simulink model "LineFollowing"  (R2013a)
settings: Solver=ode4  SolverMode=SingleTasking  StartTime=0.0  StopTime=pi  RelTol=1e-3
model workspace (MAT data in the model file):
  axleLength = Simulink.Parameter
  axleLength.Value = 9.8
  axleLength.Description = 'Distance between tire contact points
    | of the two wheels/treads
    | in units of centimeters.'
  axleLength.DataType = 'auto'
  commandPercmPerSecond = Simulink.Parameter
  commandPercmPerSecond.Value = 3.9547
  commandPercmPerSecond.Description = 'Convert units of ''command'' 
    | to units of ''cm/s''.
    | 
    | ''command'' is a value in the range [-256, 255].'
  commandPercmPerSecond.DataType = 'auto'
  symmetrizeMotors = Simulink.Parameter
  symmetrizeMotors.Value = 1
  symmetrizeMotors.Description = 'Scale one of the motor commands down 
    | (not up) to balance the motors. 
    | Once balanced, a value of x sent to either
    | motor will produce the same rate of rotation
    | in both motors.'
  symmetrizeMotors.DataType = 'auto'
  sampleTime = Simulink.Parameter
  sampleTime.Value = 0.01
  sampleTime.Description = 'Sample time (in seconds) of the trajectory simulator.'
  sampleTime.DataType = 'auto'
  commandThreshold = Simulink.Parameter
  commandThreshold.Value = 31.875
  commandThreshold.DataType = 'auto'
  plotRange = Simulink.Parameter
  plotRange.Value = 50
  plotRange.Description = 'Range of trajectory plot in units
    | of centimeters.'
  plotRange.DataType = 'auto'
libraries: ZumoBotLib x2, simulink x1
settings Model: ExtModeTrigDuration=2  Creator=pkasseba  LastModifiedBy=adesai
settings DataIOCC: SignalLoggingSaveFormat=ModelDataLogs
settings OptimizationCC: OptimizeModelRefInitCode=on  LifeSpan=1
settings DebuggingCC: SolverPrmCheckMsg=none  MultiTaskDSMMsg=warning  MultiTaskCondExecSysMsg=none  StateNameClashWarn=none  StrictBusMsg=None
settings HardwareCC: ProdBitPerInt=16  ProdBitPerPointer=8  ProdIntDivRoundTo=Zero  ProdEndianess=LittleEndian  ProdWordSize=8  ProdHWDeviceType=Atmel->AVR
settings RTWCC: SystemTargetFile=realtime.tlc  GenerateMakefile=off  TemplateMakefile=realtime.tmf  Description=Run on Target Hardware  RTWVerbose=off  ProcessScript=realtime_make_rtw_hook  IncludeERTFirstTime=on
settings STFCustomTargetCC: TargetLibSuffix=.a  GenerateSampleERTMain=on  ERTCustomFileBanners=on  SupportNonInlinedSFcns=off  SupportVariableSizeSignals=on  MATLABClassNameForMDSCustomization=Simulink.SoftwareTarget.ERTCustomization  SystemTargetFile=realtime.tlc
settings ERTTargetCC: ParMdlRefBuildCompliant=off  CompOptLevelCompliant=off  ConcurrentExecutionCompliant=off  CombineOutputUpdateFcns=off  ERTFirstTimeCompliant=off  SupportContinuousTime=on  SupportVariableSizeSignals=on  ModelStepFunctionPrototypeControlCompliant=off  CPPClassGenCompliant=off  ExtModeTransport=3  ExtModeMexFile=ext_serial_win32_comm  ExtModeMexArgs=0 1 9600  ERTSrcFileBannerTemplate=realtime_code_template.cgt  ERTHdrFileBannerTemplate=realtime_code_template.cgt  ERTDataSrcFileTemplate=realtime_code_template.cgt  ERTDataHdrFileTemplate=realtime_code_template.cgt  ERTCustomFileTemplate=realtime_file_process.tlc

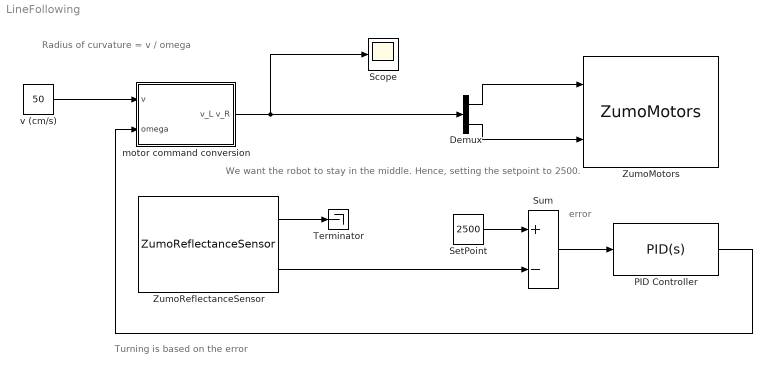
== system LineFollowing ==
  note: Turning is based on the error
  note: error
  note: We want the robot to stay in the middle. Hence,
      | setting the setpoint to 2500.
  note: Radius of curvature = v / omega
  Demux : Demux  Outputs=2
  PID Controller : simulink/Continuous/PID Controller  Controller=PID  TimeDomain=Continuous-time  SampleTime=1  IntegratorMethod=Forward Euler  FilterMethod=Forward Euler  Form=Parallel  P=0.01  I=0  D=0.005  N=1  InitialConditionSource=internal  InitialConditionForIntegrator=0  InitialConditionForFilter=0  ExternalReset=none  LimitOutput=off  UpperSaturationLimit=5  LowerSaturationLimit=-5  LinearizeAsGain=on  AntiWindupMode=none  Kb=1  TrackingMode=off  Kt=1  PParamMin=[]  PParamMax=[]  IParamMin=[]  IParamMax=[]  DParamMin=[]  DParamMax=[]  NParamMin=[]  NParamMax=[]  KbParamMin=[]  KbParamMax=[]  KtParamMin=[]  KtParamMax=[]  POutMin=[]  POutMax=[]  IOutMin=[]  IOutMax=[]  DOutMin=[]  DOutMax=[]  NOutMin=[]  NOutMax=[]  KbOutMin=[]  KbOutMax=[]  KtOutMin=[]  KtOutMax=[]  IntegratorOutMin=[]  IntegratorOutMax=[]  FilterOutMin=[]  FilterOutMax=[]  SumOutMin=[]  SumOutMax=[]  SumI1OutMin=[]  SumI1OutMax=[]  SumI2OutMin=[]  SumI2OutMax=[]  SumI3OutMin=[]  SumI3OutMax=[]  SumDOutMin=[]  SumDOutMax=[]  SaturationOutMin=[]  SaturationOutMax=[]  IntegratorContinuousStateAttributes=''  IntegratorStateMustResolveToSignalObject=off  IntegratorRTWStateStorageClass=Auto  FilterContinuousStateAttributes=''  FilterStateMustResolveToSignalObject=off  FilterRTWStateStorageClass=Auto
  Scope : Scope
  SetPoint : Constant  Value=2500
  Sum : Sum  Inputs=+-
  Terminator : Terminator
  ZumoMotors : ZumoBotLib/ZumoMotors  flipLeft=off  flipRight=off
  ZumoReflectanceSensor : ZumoBotLib/ZumoReflectanceSensor  sampleTime_dd=sampleTime  emitterPin_dd=255  debug_dd=off
  motor command conversion : Subsystem
  v (cm/s) : Constant  Value=50  SampleTime=sampleTime
  wires:
  v (cm/s)/1 -> motor command conversion/1(v)
  motor command conversion/1(v_L v_R) -> Scope/1, Demux/1
  Demux/1 -> ZumoMotors/1
  Demux/2 -> ZumoMotors/2
  ZumoReflectanceSensor/1 -> Terminator/1
  ZumoReflectanceSensor/2 -> Sum/2
  SetPoint/1 -> Sum/1
  Sum/1 -> PID Controller/1
  PID Controller/1 -> motor command conversion/2(omega)

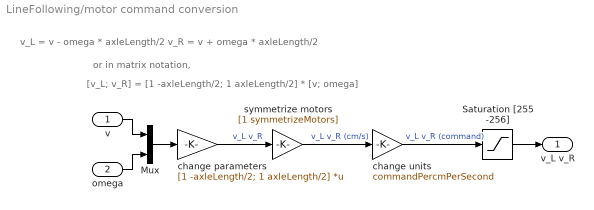
== system LineFollowing/motor command conversion ==
  note: or in matrix notation,
  note: v_L  = v - omega * axleLength/2
      | v_R = v + omega * axleLength/2
  note: [v_L; v_R] = [1 -axleLength/2; 1 axleLength/2] * [v; omega]
  v : Inport
  omega : Inport  Port=2
  Mux : Mux  Inputs=2
  Saturation [255 -256] : Saturate  UpperLimit=255  LowerLimit=-256
  change parameters : Gain  Gain=[1 -axleLength/2; 1 axleLength/2]  Multiplication=Matrix(K*u)
  change units : Gain  Gain=commandPercmPerSecond
  symmetrize motors : Gain  Gain=[1 symmetrizeMotors]
  v_L v_R : Outport
  wires:
  change parameters/1 -> symmetrize motors/1  "v_L v_R"
  change units/1 -> Saturation [255 -256]/1  "v_L v_R (command)"
  symmetrize motors/1 -> change units/1  "v_L v_R (cm/s)"
  Saturation [255 -256]/1 -> v_L v_R/1
  Mux/1 -> change parameters/1
  omega/1 -> Mux/2
  v/1 -> Mux/1
